simulink model "firstsimulink"  (R2018a)
settings: Solver=VariableStepAuto  StartTime=0.0  StopTime=1  RelTol=1e-3
libraries: simulink x2, dspsnks4 x1, dspspect3 x1
settings Model: Creator=wardzin3  LastModifiedBy=wardzin3

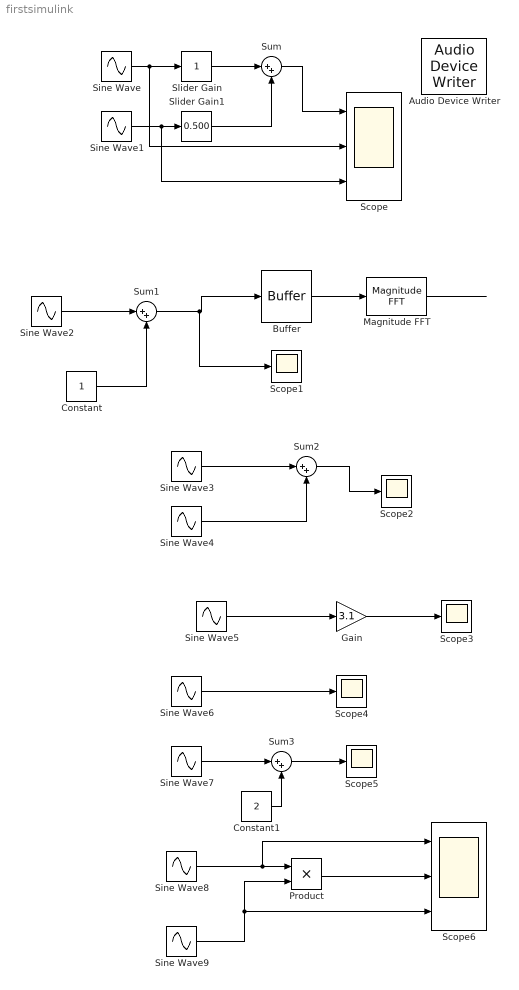
== system firstsimulink ==
  Audio Device Writer : dspsnks4/Audio Device Writer  Driver=ALSA  Device=Default  InheritSampleRate=on  SampleRate=44100  BitDepth=16-bit integer  BufferSize=4096  NumBuffers=10  DefaultOutputChannelMapping=on  OutputChannelMapping=1:2  OutputNumUnderrunSamples=off  DriverIdx=8  DeviceWarnFlag=''
  Buffer : Buffer  N=256  OutputFrames=off
  Constant : Constant
  Constant1 : Constant  Value=2
  Gain : Gain  Gain=3.1
  Magnitude FFT : dspspect3/Magnitude FFT  mag_or_magsq=Magnitude squared  FFTImplementation=Auto  fftLenInherit=off  fftsize=256  WrapInput=on
      settings: SourceProductName=DSP System Toolbox  SourceProductBaseCode=DS
  Product : Product
  Scope : Scope  NumInputPorts=3
  Scope{1..5} (5 alike) : Scope
  Scope6 : Scope  NumInputPorts=3
  Sine Wave{,3,6..7} (4 alike) : Sin  Frequency=1000*2*pi  Samples=2*pi/(1000)  SampleTime=1/48000
  Sine Wave1 : Sin  Frequency=2000*2*pi  SampleTime=1/48000
  Sine Wave2 : Sin  SineType=Sample based  Samples=48  SampleTime=1/48000
  Sine Wave4 : Sin  Amplitude=1/2  Frequency=2000*2*pi  Samples=2*pi/(1000)  SampleTime=1/48000
  Sine Wave5 : Sin  Frequency=500/pi  Samples=2*pi/(1000)  SampleTime=1/48000
  Sine Wave8 : Sin  Frequency=500*2*pi  Samples=2*pi/(1000)  SampleTime=1/48000
  Sine Wave9 : Sin  Frequency=31.25*2*pi  Samples=2*pi/(1000)  SampleTime=1/48000
  Slider Gain : simulink/Math Operations/Slider Gain  gain=1  low=0  high=2
  Slider Gain1 : simulink/Math Operations/Slider Gain  gain=0.500  low=0  high=1
  Sum{,1..3} (4 alike) : Sum  Inputs=|++
  wires:
  Sum/1 -> Scope/1
  Sine Wave/1 -> Scope/2, Slider Gain/1
  Slider Gain/1 -> Sum/1
  Sine Wave1/1 -> Scope/3, Slider Gain1/1
  Slider Gain1/1 -> Sum/2
  Sine Wave2/1 -> Sum1/1
  Constant/1 -> Sum1/2
  Magnitude FFT/1 -> ?
  Buffer/1 -> Magnitude FFT/1
  Sum1/1 -> Scope1/1, Buffer/1
  Sine Wave3/1 -> Sum2/1
  Sine Wave4/1 -> Sum2/2
  Sum2/1 -> Scope2/1
  Sine Wave5/1 -> Gain/1
  Gain/1 -> Scope3/1
  Sine Wave6/1 -> Scope4/1
  Sum3/1 -> Scope5/1
  Sine Wave7/1 -> Sum3/1
  Constant1/1 -> Sum3/2
  Sine Wave8/1 -> Product/1, Scope6/1
  Sine Wave9/1 -> Product/2, Scope6/3
  Product/1 -> Scope6/2
